simulink model "TestStruct"  (R2018a)
settings: Solver=ode4  StartTime=0.0  StopTime=10  FixedStep=0.1  RelTol=1e-3  EnableMultiTasking=on
settings Model: SimulationMode=accelerator  EnablePacing=on  Creator=Hungs  LastModifiedBy=Hungs

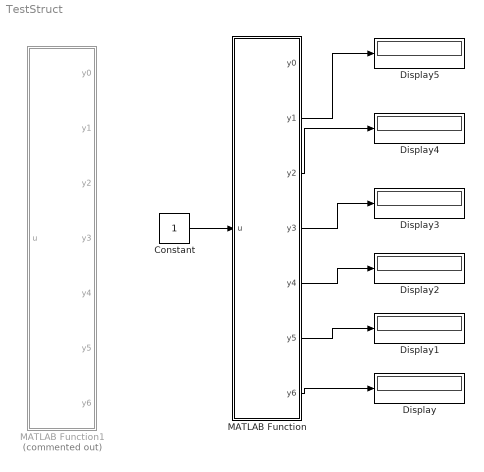
== system TestStruct ==
  Constant : Constant
  Display{,1..5} (6 alike) : Display
      settings: Decimation=2
  MATLAB Function : MATLAB Function  TreatAsAtomicUnit=on
  MATLAB Function1 : MATLAB Function  Commented=on  TreatAsAtomicUnit=on
  wires:
  MATLAB Function/2(y1) -> Display5/1
  Constant/1 -> MATLAB Function/1(u)
  MATLAB Function/3(y2) -> Display4/1
  MATLAB Function/4(y3) -> Display3/1
  MATLAB Function/5(y4) -> Display2/1
  MATLAB Function/6(y5) -> Display1/1
  MATLAB Function/7(y6) -> Display/1

== matlab function TestStruct/MATLAB Function ==
  data: y0 output; u input; y1 output; y2 output; y3 output; y4 output; y5 output; y6 output
function [y0, y1,y2,y3,y4,y5,y6] = fcn(u)
if u==1
    y0 = evalin('base','value0');
    y1 = evalin('base','value0');
    y2 = evalin('base','value0');
    y3 = evalin('base','value0');
    y4 = evalin('base','value0');
    y5 = evalin('base','value0');
    y6 = evalin('base','value0');
end
end

== matlab function TestStruct/MATLAB Function1 ==
  data: y0 output; u input; y1 output; y2 output; y3 output; y4 output; y5 output; y6 output
function [y0, y1,y2,y3,y4,y5,y6] = fcn(u)
coder.extrinsic('AdsReadStruct');
y0 = double(0);
y1 = double(0);
y2 = double(0);
y3 = double(0);
y4 = double(0);
y5 = double(0);
y6 = double(0);
if u==1
    [y0, y1, y2, y3, y4, y5, y6] = AdsReadStruct();
end
end
